simulink model "Auxiliaries_Control"  (R2016b)
settings: Solver=FixedStepDiscrete  StartTime=0.0  StopTime=inf  FixedStep=AuxCtrl.tiSimnTiStep_C.Value  RelTol=1e-3  EnableMultiTasking=on
settings Model: Creator=djuenema  LastModifiedBy=djuenema
settings DataIOCC: SaveFormat=StructureWithTime  SaveOutput=off  DSMLogging=off  VisualizeSimOutput=off  SaveTime=off  SignalLoggingName=Results
settings OptimizationCC: BlockReduction=off  ConditionallyExecuteInputs=off  LifeSpan=inf
settings DebuggingCC: AllowSymbolicDim=off  SFUnexpectedBacktrackingDiag=warning  SFNoUnconditionalDefaultTransitionDiag=warning  SFExecutionAtInitializationDiag=none
settings ModelReferenceCC: ModelReferenceNumInstancesAllowed=Single  PropagateSignalLabelsOutOfModel=off
settings GRTTargetCC: TargetLangStandard=C89/C90 (ANSI)
settings ConfigComp: CovMetricSettings=dw  CovHtmlReporting=on  CovSaveCumulativeToWorkspaceVar=on  CovSaveSingleToWorkspaceVar=on  CovExternalEMLEnable=off

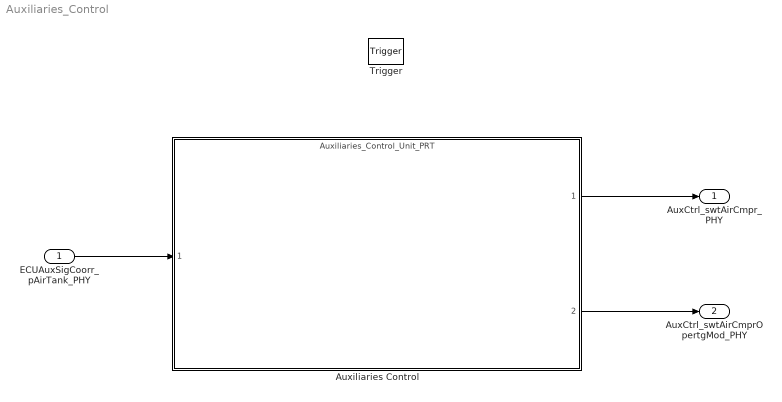
== system Auxiliaries_Control ==
  ECUAuxSigCoorr_pAirTank_PHY : Inport
  Trigger : TriggerPort  TriggerType=function-call  VariantControl=Variant  PortDimensions=1
  Auxiliaries Control : ModelReference  ModelNameDialog=Auxiliaries_Control_Unit_PRT.slxp  ModelReferenceVersion=1.52  CopyOfModelProtected=on
  AuxCtrl_swtAirCmpr_PHY : Outport
  AuxCtrl_swtAirCmprOpertgMod_PHY : Outport  Port=2
  wires:
  Auxiliaries Control/2 -> AuxCtrl_swtAirCmprOpertgMod_PHY/1
  Auxiliaries Control/1 -> AuxCtrl_swtAirCmpr_PHY/1
  ECUAuxSigCoorr_pAirTank_PHY/1 -> Auxiliaries Control/1
